simulink model "ee105lab4part1"  (R2016b)
settings: Solver=VariableStepAuto  StartTime=0.0  StopTime=1000.0  RelTol=1e-3
settings Model: Creator=jesselayman  LastModifiedBy=jesselayman

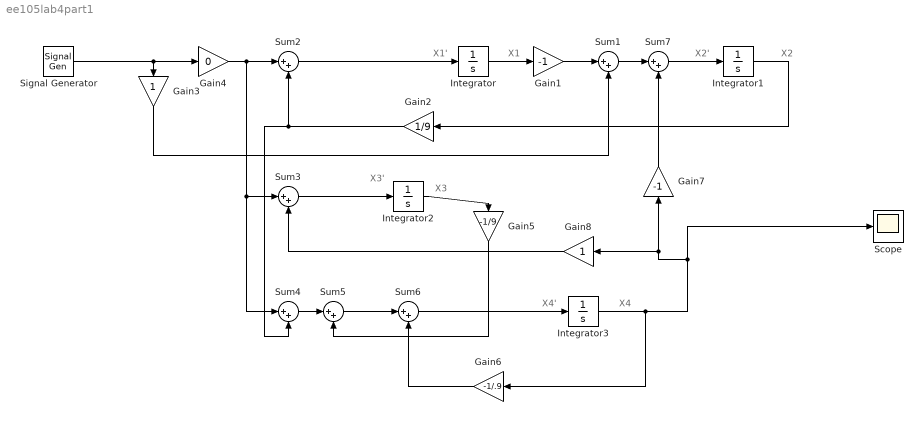
== system ee105lab4part1 ==
  note: X4'
  note: X3'
  note: X1
  note: X1'
  note: X2'
  note: X2
  note: X3
  note: X4
  Gain1 : Gain  Gain=-1
  Gain2 : Gain  Gain=1/9
  Gain3 : Gain
  Gain4 : Gain  Gain=0
  Gain5 : Gain  Gain=-1/9
  Gain6 : Gain  Gain=-1/.9
  Gain7 : Gain  Gain=-1
  Gain8 : Gain
  Integrator{,1..3} (4 alike) : Integrator
  Scope : Scope
  Signal Generator : SignalGenerator  Frequency=1000
  Sum{1..7} (7 alike) : Sum  Inputs=|++
  wires:
  Integrator1/1 -> Gain2/1
  Integrator/1 -> Gain1/1
  Signal Generator/1 -> Gain4/1, Gain3/1
  Gain3/1 -> Sum1/2
  Gain1/1 -> Sum1/1
  Gain4/1 -> Sum4/1, Sum3/1, Sum2/1
  Sum2/1 -> Integrator/1
  Gain2/1 -> Sum4/2, Sum2/2
  Sum3/1 -> Integrator2/1
  Integrator3/1 -> Gain6/1, Scope/1, Gain8/1, Gain7/1
  Sum4/1 -> Sum5/1
  Integrator2/1 -> Gain5/1
  Gain5/1 -> Sum5/2
  Sum5/1 -> Sum6/1
  Sum6/1 -> Integrator3/1
  Gain6/1 -> Sum6/2
  Sum1/1 -> Sum7/1
  Sum7/1 -> Integrator1/1
  Gain7/1 -> Sum7/2
  Gain8/1 -> Sum3/2
